simulink model "model_bicycleRider.slx"  (R2019b)
settings: Solver=VariableStepAuto  StartTime=0.0  StopTime=15.84  RelTol=1e-3
undefined symbols (not defined in the file): magnitude
libraries: SignalEditorBlockLib x1
settings Model: Creator=rosswilkinson  LastModifiedBy=rosswilkinson
settings DataIOCC: InspectSignalLogs=on

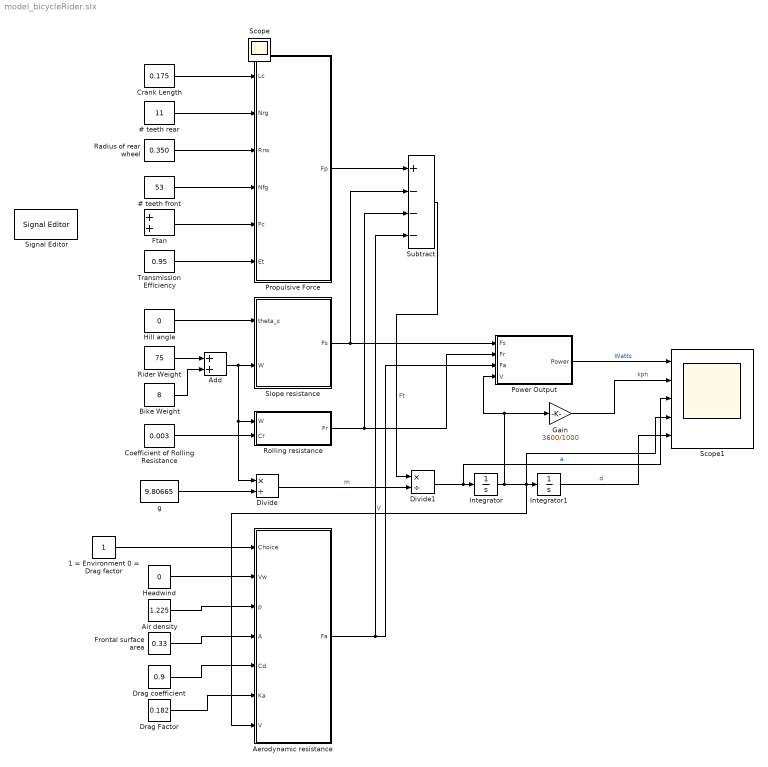
== system model_bicycleRider.slx ==
  " Drag coefficient" : Constant  Value=0.9
  # teeth front : Constant  Value=53
  # teeth rear : Constant  Value=11
  1 = Environment 0 = Drag factor : Constant
  Add : Sum
  Aerodynamic resistance : Subsystem
  Air density : Constant  Value=1.225
  "Bike Weight " : Constant  Value=8
  Coefficient of Rolling Resistance : Constant  Value=0.003
  Crank Length : Constant  Value=0.175
  Divide : Product  Inputs=*/
  Divide1 : Product  Inputs=*/
  Drag Factor : Constant  Value=0.182
  Frontal surface area : Constant  Value=0.33
  Ftan : Sum
  Gain : Gain  Gain=3600/1000
  Headwind : Constant  Value=0
  "Hill angle " : Constant  Value=0
  Integrator : Integrator
  Integrator1 : Integrator
  Power Output : Subsystem
  Propulsive Force : Subsystem
  Radius of rear wheel : Constant  Value=0.350
  "Rider Weight " : Constant  Value=75
  Rolling resistance : Subsystem
  Scope1 : Scope  NumInputPorts=5
  Signal Editor : SignalEditorBlockLib/Signal Editor  FileName=untitled.mat  ActiveScenario=Scenario  ActiveSignal=Signal 1  IsBus=off  OutputBusObjectStr=Bus: BusObject  SampleTime=0  Interpolate=off  ZeroCross=off  OutputAfterFinalValue=Setting to zero  Unit=inherit  PreserveSignalName=on
      settings: SourceProductName=Simulink
  Slope resistance : Subsystem
  Subtract : Sum  Inputs=+---
  Transmission Efficiency : Constant  Value=0.95
  g : Constant  Value=9.80665
  Scope : Scope
  wires:
  # teeth rear/1 -> Propulsive Force/2("Nrg ")
  "Rider Weight "/1 -> Add/1
  Crank Length/1 -> Propulsive Force/1("Lc ")
  # teeth front/1 -> Propulsive Force/4("Nfg ")
  Radius of rear wheel/1 -> Propulsive Force/3("Rrw ")
  "Bike Weight "/1 -> Add/2
  Add/1 -> Divide/1, Rolling resistance/1("W "), Slope resistance/2("W ")
  Coefficient of Rolling Resistance/1 -> Rolling resistance/2("Cr ")
  Ftan/1 -> Propulsive Force/5("Fc ")
  Transmission Efficiency/1 -> Propulsive Force/6(Et)
  "Hill angle "/1 -> Slope resistance/1(theta_s)
  g/1 -> Divide/2
  1 = Environment 0 = Drag factor/1 -> Aerodynamic resistance/1(Choice)
  Headwind/1 -> Aerodynamic resistance/2(Vw)
  Air density/1 -> Aerodynamic resistance/3(p)
  Frontal surface area/1 -> Aerodynamic resistance/4(A)
  " Drag coefficient"/1 -> Aerodynamic resistance/5(Cd)
  Drag Factor/1 -> Aerodynamic resistance/6(Ka)
  Propulsive Force/1("Fp ") -> Subtract/1
  Slope resistance/1(Fs) -> Power Output/1(Fs), Subtract/2
  Rolling resistance/1("Fr ") -> Power Output/2(Fr), Subtract/3
  Aerodynamic resistance/1(Fa) -> Power Output/3(Fa), Subtract/4
  Divide/1 -> Divide1/2  "m"
  Subtract/1 -> Divide1/1  "Ft"
  Divide1/1 -> Scope1/3, Integrator/1  "a"
  Integrator/1 -> Scope1/4, Aerodynamic resistance/7(V), Integrator1/1, Power Output/4(V), Gain/1  "V"
  Power Output/1(Power) -> Scope1/1  "Watts"
  Gain/1 -> Scope1/2  "kph"
  Integrator1/1 -> Scope1/5  "d"

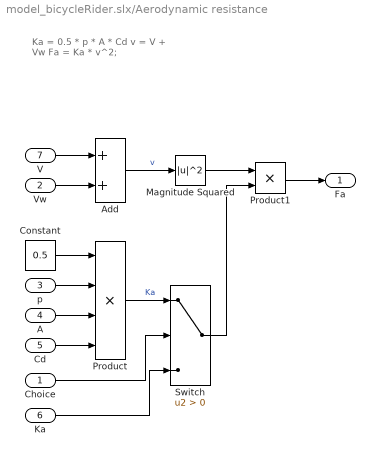
== system model_bicycleRider.slx/Aerodynamic resistance ==
  note: Ka = 0.5 * p * A * Cd
      |
      | v = V + Vw
      |
      | Fa = Ka * v^2;
  Choice : Inport
  Vw : Inport  Port=2
  p : Inport  Port=3
  A : Inport  Port=4
  Cd : Inport  Port=5
  Ka : Inport  Port=6
  V : Inport  Port=7
  Add : Sum
  Constant : Constant  Value=0.5
  Magnitude Squared : Math  Operator=magnitude^2  SignedPower=off  SaturateOnIntegerOverflow=on
  Product : Product  Inputs=4
  Product1 : Product
  Switch : Switch  Criteria=u2 > Threshold
  Fa : Outport
  wires:
  Constant/1 -> Product/1
  A/1 -> Product/3
  Product/1 -> Switch/1  "Ka"
  Cd/1 -> Product/4
  p/1 -> Product/2
  V/1 -> Add/1
  Add/1 -> Magnitude Squared/1  "v"
  Vw/1 -> Add/2
  Product1/1 -> Fa/1
  Magnitude Squared/1 -> Product1/1
  Choice/1 -> Switch/2
  Switch/1 -> Product1/2
  Ka/1 -> Switch/3

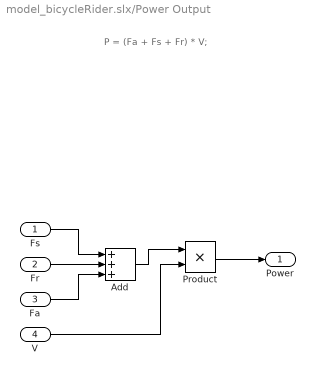
== system model_bicycleRider.slx/Power Output ==
  note: P = (Fa + Fs + Fr) * V;
  Fs : Inport
  Fr : Inport  Port=2
  Fa : Inport  Port=3
  V : Inport  Port=4
  Add : Sum  Inputs=+++
  Product : Product
  Power : Outport
  wires:
  Fs/1 -> Add/1
  Fr/1 -> Add/2
  Fa/1 -> Add/3
  V/1 -> Product/2
  Add/1 -> Product/1
  Product/1 -> Power/1

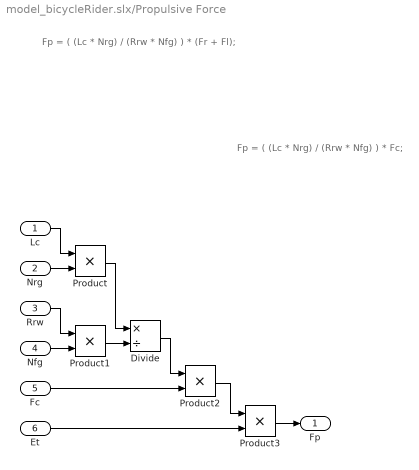
== system model_bicycleRider.slx/Propulsive Force ==
  note: Fp = ( (Lc * Nrg) / (Rrw * Nfg) ) * Fc;
  note: Fp = ( (Lc * Nrg) / (Rrw * Nfg) ) * (Fr + Fl);
  "Lc " : Inport
  "Nrg " : Inport  Port=2
  "Rrw " : Inport  Port=3
  "Nfg " : Inport  Port=4
  "Fc " : Inport  Port=5
  Et : Inport  Port=6
  Divide : Product  Inputs=*/
  Product{,1..3} (4 alike) : Product
  "Fp " : Outport
  wires:
  "Lc "/1 -> Product/1
  "Nrg "/1 -> Product/2
  "Rrw "/1 -> Product1/1
  "Nfg "/1 -> Product1/2
  Product/1 -> Divide/1
  Product1/1 -> Divide/2
  Divide/1 -> Product2/1
  "Fc "/1 -> Product2/2
  Product3/1 -> "Fp "/1
  Et/1 -> Product3/2
  Product2/1 -> Product3/1

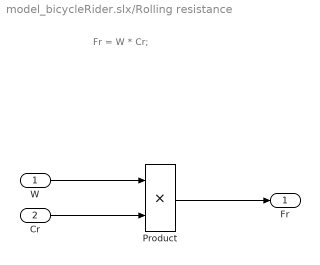
== system model_bicycleRider.slx/Rolling resistance ==
  note: Fr = W * Cr;
  "W " : Inport
  "Cr " : Inport  Port=2
  Product : Product
  "Fr " : Outport
  wires:
  "W "/1 -> Product/1
  "Cr "/1 -> Product/2
  Product/1 -> "Fr "/1

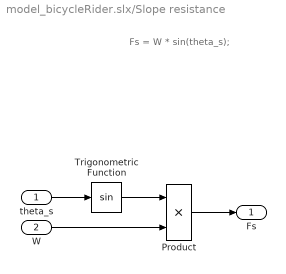
== system model_bicycleRider.slx/Slope resistance ==
  note: Fs = W * sin(theta_s);
  theta_s : Inport
  "W " : Inport  Port=2
  Product : Product
  Trigonometric Function : Trigonometry
  Fs : Outport
  wires:
  Product/1 -> Fs/1
  theta_s/1 -> Trigonometric Function/1
  Trigonometric Function/1 -> Product/1
  "W "/1 -> Product/2
